simulink model "Simulink_PID_Plant"  (R2021a)
settings: Solver=VariableStepAuto  StartTime=0.0  StopTime=10.0  RelTol=1e-3
libraries: simulink x1
settings Model: Creator=gino  LastModifiedBy=gino

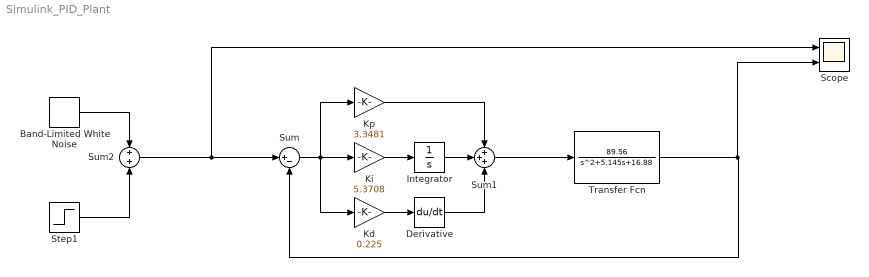
== system Simulink_PID_Plant ==
  Band-Limited White Noise : simulink/Sources/Band-Limited White Noise  Cov=[0]  Ts=0.01  seed=[23341]
  Derivative : Derivative
  Integrator : Integrator
  Kd : Gain  Gain=0.225
  Ki : Gain  Gain=5.3708
  Kp : Gain  Gain=3.3481
  Scope : Scope  NumInputPorts=2
  Step1 : Step  Time=0.01  After=25  SampleTime=0.01
  Sum : Sum  Inputs=|+-
  Sum1 : Sum  Inputs=+++
  Sum2 : Sum
  Transfer Fcn : TransferFcn  Numerator=[89.56]  Denominator=[1 5.145 16.88]
  wires:
  Sum2/1 -> Scope/1, Sum/1
  Sum/1 -> Kd/1, Ki/1, Kp/1
  Kd/1 -> Derivative/1
  Ki/1 -> Integrator/1
  Kp/1 -> Sum1/1
  Integrator/1 -> Sum1/2
  Derivative/1 -> Sum1/3
  Sum1/1 -> Transfer Fcn/1
  Transfer Fcn/1 -> Scope/2, Sum/2
  Band-Limited White Noise/1 -> Sum2/1
  Step1/1 -> Sum2/2
